simulink model "Arduino_PID_Interface"  (R2019b)
settings: Solver=VariableStepAuto  StartTime=0.0  StopTime=inf  RelTol=1e-3
undefined symbols (not defined in the file or in its folder): __PRM__SERIALIZED__DATA__, LF, serial, SubsystemReferenceBlock
libraries: instrumentlib x3
settings Model: Creator=VM  LastModifiedBy=VM

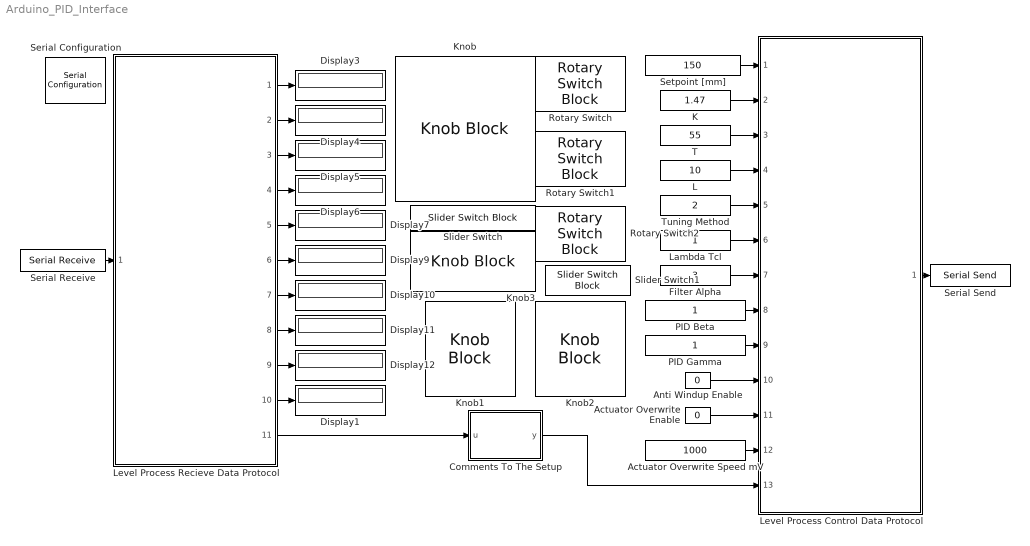
== system Arduino_PID_Interface ==
  Actuator Overwrite Enable : Constant  Value=0  OutDataTypeStr=uint8
  Actuator Overwrite Speed mV : Constant  Value=1000  OutDataTypeStr=double
  Anti Windup Enable : Constant  Value=0  OutDataTypeStr=uint8
  Comments To The Setup : MATLAB Function  TreatAsAtomicUnit=on
  Display{1,3..7,9..12} (10 alike) : Display
  Filter Alpha : Constant  Value=3
  K : Constant  Value=1.47
  Knob : KnobBlock  ScaleMax=300
  Knob1 : KnobBlock  ScaleMax=1
  Knob2 : KnobBlock  ScaleMax=1
  Knob3 : KnobBlock  ScaleMax=5000
  L : Constant  Value=10
  Lambda Tcl : Constant
  Level Process Control Data Protocol : Subsystem  BlockKeywords=__PRM__SERIALIZED__DATA__:SubsystemReferenceBlock  ReferencedSubsystem=ControlSample
  Level Process Recieve Data Protocol : Subsystem  BlockKeywords=__PRM__SERIALIZED__DATA__:SubsystemReferenceBlock  ReferencedSubsystem=DataSample
  PID Beta : Constant
  PID Gamma : Constant
  Rotary Switch : RotarySwitchBlock
      settings: Values={{'AMIGO PI', 'AMIGO PID', 'Lambda PI', 'Lambda PID', 'SIMC PI', 'SIMC PID'}, [1 2 3 4 5 6]}
  Rotary Switch1 : RotarySwitchBlock
      settings: Values={{'L', 'T', '3T'}, [1 2 3]}
  Rotary Switch2 : RotarySwitchBlock
      settings: Values={{'Bypass', '0.01', '0.02', '0.03', '0.04', '0.05'}, [0 1 2 3 4 5]}
  Serial Configuration : instrumentlib/Serial Configuration  Priority=-200000  ComPortMenu=<Please select a port...>  ComPort=COM3  ObjConstructor=serial('COM3');  BaudRate=115200  DataBits=8  Parity=none  StopBits=1  FlowControl=none  Timeout=10  ByteOrder=LittleEndian
  Serial Receive : instrumentlib/Serial Receive  ComPortMenu=<Please select a port...>  ComPort=COM3  ObjConstructor=serial('COM3');  Header=<D>  Terminator=LF ('\n')  DataSize="[1  32]"  DataType=uint8  EnableBlockingMode=on  ActionDataUnavailable=Output last received value  CustomValue=0  SampleTime=0.001
  Serial Send : instrumentlib/Serial Send  ComPortMenu=<Please select a port...>  ComPort=COM3  ObjConstructor=serial('COM3');  Header=<C>  Terminator=LF ('\n')  EnableBlockingMode=on
  Setpoint [mm] : Constant  Value=150  OutDataTypeStr=uint16
  Slider Switch : SliderSwitchBlock
      settings: Values={{'Off', 'On'}, [0 1]}
  Slider Switch1 : SliderSwitchBlock
      settings: Values={{'Off', 'On'}, [0 1]}
  T : Constant  Value=55
  Tuning Method : Constant  Value=2
  wires:
  Serial Receive/1 -> Level Process Recieve Data Protocol/1
  Setpoint [mm]/1 -> Level Process Control Data Protocol/1
  Level Process Recieve Data Protocol/1 -> Display3/1
  Level Process Recieve Data Protocol/2 -> Display4/1
  Level Process Recieve Data Protocol/3 -> Display5/1
  Level Process Recieve Data Protocol/4 -> Display6/1
  Level Process Recieve Data Protocol/5 -> Display7/1
  Level Process Recieve Data Protocol/6 -> Display9/1
  Level Process Recieve Data Protocol/7 -> Display10/1
  Level Process Recieve Data Protocol/8 -> Display11/1
  Level Process Recieve Data Protocol/9 -> Display12/1
  Tuning Method/1 -> Level Process Control Data Protocol/5
  Filter Alpha/1 -> Level Process Control Data Protocol/7
  Level Process Control Data Protocol/1 -> Serial Send/1
  K/1 -> Level Process Control Data Protocol/2
  PID Beta/1 -> Level Process Control Data Protocol/8
  PID Gamma/1 -> Level Process Control Data Protocol/9
  T/1 -> Level Process Control Data Protocol/3
  L/1 -> Level Process Control Data Protocol/4
  Lambda Tcl/1 -> Level Process Control Data Protocol/6
  Level Process Recieve Data Protocol/11 -> Comments To The Setup/1(u)
  Comments To The Setup/1(y) -> Level Process Control Data Protocol/13
  Level Process Recieve Data Protocol/10 -> Display1/1
  Actuator Overwrite Speed mV/1 -> Level Process Control Data Protocol/12
  Actuator Overwrite Enable/1 -> Level Process Control Data Protocol/11
  Anti Windup Enable/1 -> Level Process Control Data Protocol/10

== matlab function Arduino_PID_Interface/Comments To The Setup ==
  data: u input; y output
% DHBW Mosbach
% Mechatronische Systeme 4
% Dr.-Ing. Vanessa Romero Segovia
% MT17B Gruppe 3 (Sarah Plieninger, Fabian Redaoui, Raphael Kuttruf)

function y = fcn(u)

% Actuator overwrite can be used to measure the Step Response

% Gamma is only applied if the Filter is on Bypass

% If Time Sync is connected a CntrolSample is send 
% every Time an new DataSample arrives
% If A Zero Order Hold block is needed 
% in front of the Serial Send Block if you want to send 
% a Control Sample every X-times a DataSample arrives

%  Dont use the INT De-/Serialize Blocks ! They don't work correctly 
% Serializing signed and unsigned integers at the same time is not so easy

y = u;
